simulink library "pmm"  (R2021b)
settings: Solver=VariableStepAuto  StartTime=0.0  StopTime=10.0  RelTol=1e-3
undefined symbols (not defined in the file or in its folder): ENUM_ACMAINRLYSTS_OPEN, ENUM_ACPRECHRGRLYSTS_OPEN, ENUM_B2VRLYSTA_OPEN, ENUM_BMSHVSTS_HVOPEN, ENUM_BRAKEPEDAL_RELEASED, ENUM_CACRLYDEM_CLOSE, ENUM_CACRLYSTS_OPEN, ENUM_CHRGFAULT_ACRLYFAIL, ENUM_CHRGFAULT_BCUHVFAIL, ENUM_CHRGFAULT_BCUNEGFAIL, ENUM_CHRGFAULT_BCUTIMEOUT, ENUM_CHRGFAULT_DCDCENABLE, ENUM_CHRGFAULT_DCDCRLYFAIL, ENUM_CHRGFAULT_HVILFAIL, ENUM_CHRGFAULT_PDUHVFAIL, ENUM_CHRGFAULT_RLYCHKFAIL, ENUM_DCDCEACPCURLYSTA_CLOSED, ENUM_DCDCEACPCURLYSTA_FAILTOCLOSE, ENUM_DCDCEACPCURLYSTA_OPEN, ENUM_DCDCEACPCURLYSTA_WELDED, ENUM_DCDCENABLESTS_READY, ENUM_DCDCRLYSTS_OPEN, ENUM_EHPSRLYDEM_CLOSE, ENUM_EHPSRLYSTS_OPEN, ENUM_FOGRLYENCMD_DISABLE, ENUM_GEARACTUALPOSN_D, ENUM_HVPWROFFREQ_POWEROFF, ENUM_KEYSTATUS_OFF, ENUM_KEYSTATUS_ON, ENUM_KEYSTATUS_START, ENUM_LOWBATTVOLTAGE_NORMAL, ENUM_LOWBATTVOLTAGE_POWERDOWN, ENUM_LOWBATTVOLTAGE_POWERUP, ENUM_MCUHVLOOP_POWEROFF, ENUM_MCUHVLOOPSTS_OPEN, ENUM_MCUMAINRLYSTS_OPEN, ENUM_MCUPRECHRGRLYSTS_OPEN, ENUM_PDFAULT_ACRLYOPEN, ENUM_PDFAULT_BCUDISABLE, ENUM_PDFAULT_DCDCDISABLE, ENUM_PDFAULT_DCDCRLYOPEN, ENUM_PDFAULT_EACDISABLE, ENUM_PDFAULT_EACRLYOPEN, ENUM_PDFAULT_EHPSDISABLE, ENUM_PDFAULT_EHPSRLYOPEN, ENUM_PDFAULT_MCUDISABLE, ENUM_PDFAULT_MCUDISCHRG, ENUM_PDFAULT_MCURLYOPEN, ENUM_PEUSELFCHKSTS_NOFAULT, ENUM_PLUGINSTS_NOPLUGIN, ENUM_PLUGINSTS_PLUGIN, ENUM_PMMMODE_DRIVE, ENUM_PMMMODE_LVBATCHRG, ENUM_PUSTATE_DCDCENABLE, ENUM_PUSTATE_EACPRESCHECK, ENUM_PUSTATE_EHPSENABLE, ENUM_PUSTATE_MCUENABLE, ENUM_PUSTATE_PDUMCURLYCLOSED, ENUM_PUSTATE_POWERUPFAIL, ENUM_TARGETGEAR_REVERSE ... (+126)
libraries: hcu_lib x45, simulink x5, ddm x1, dsc x1
(part 2 of 7)

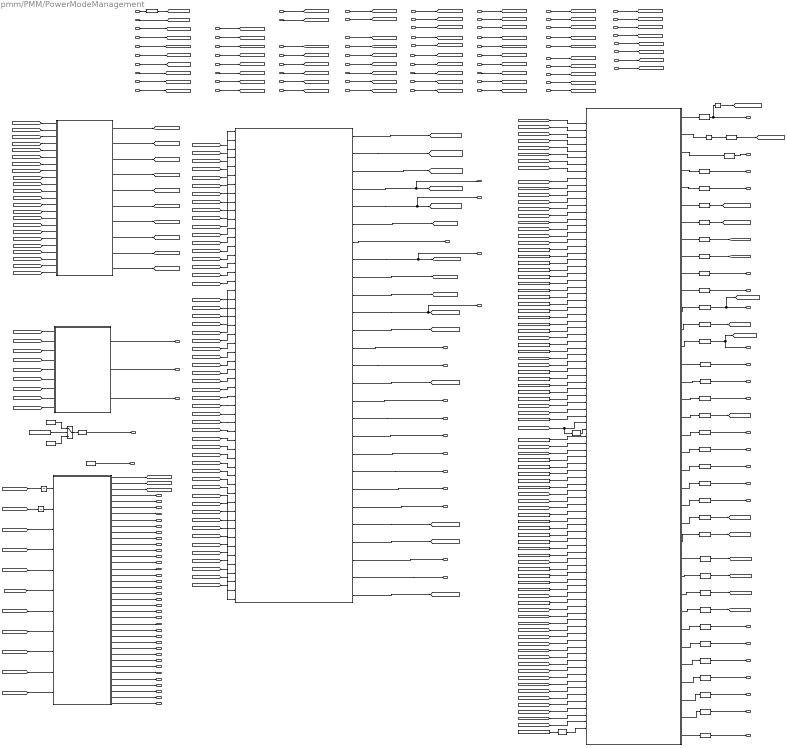
== system pmm/PMM/PowerModeManagement ==
  note: BDDM_outputs
  note: BDDM_outputs
  note: DDM_outpus
  note: BAPP_outputs
  note: BAPP_outputs
  note: BAPP_outputs
  note: BAPP_outputs
  note: BAPP_outputs
  note: BACC_outputs
  note: BVPSA_outputs
  task_time_s : Inport
  VPSA_Keystatus_enum : Inport  Port=2
  VPSA_EmergencyShutDown_flg : Inport  Port=3
  VPSA_AlcLockPass_flg : Inport  Port=4
  VACC_CACPresReady_flg : Inport  Port=5
  VTHC_AfterrunningMode_flg : Inport  Port=6
  VINP_DCChrgConnectSts_enum : Inport  Port=7
  VINP_BMSHVSts_enum : Inport  Port=8
  VINP_HVPwrOffReq_enum : Inport  Port=9
  VINP_MCUInVol_V : Inport  Port=10
  VINP_BMSChrgStatus_enum : Inport  Port=11
  VINP_B2VFaultCode_enum : Inport  Port=12
  VINP_AtvDisChgEnFbk_flg : Inport  Port=13
  VINP_MCUIGBTEnFbk_flg : Inport  Port=14
  VINP_MCUFailGrade_enum : Inport  Port=15
  VINP_MCUFailCode_enum : Inport  Port=16
  VINP_B2VHVILFault_flg : Inport  Port=17
  VINP_B2VMainNegRlySta_enum : Inport  Port=18
  VINP_B2VDCChgP1RlySta_enum : Inport  Port=19
  VINP_B2VDCChgN1RlySta_enum : Inport  Port=20
  VINP_B2VSOC_pct : Inport  Port=21
  VINP_MotorSpd_rpm : Inport  Port=22
  VINP_B2VPackCurr_A : Inport  Port=23
  VINP_B2VPackInsideVol_V : Inport  Port=24
  VINP_EACEnSta_enum : Inport  Port=25
  VINP_EHPSEnableStstus_enum : Inport  Port=26
  VINP_MCUHVLoopSts_enum : Inport  Port=27
  VINP_DCDCEnableStstus_enum : Inport  Port=28
  VINP_DCDCEnSta_enum : Inport  Port=29
  VINP_DCDCOutVol_V : Inport  Port=30
  VINP_PEUSelfChkSts_enum : Inport  Port=31
  VINP_MCUPrechrgRlySts_enum : Inport  Port=32
  VINP_HVILSta_enum : Inport  Port=33
  VINP_PDUMCUPosRlySta_enum : Inport  Port=34
  VINP_PDUACRlySta_enum : Inport  Port=35
  VINP_PDU3in1RlySta_enum : Inport  Port=36
  VINP_ParkBrakeSW_flg : Inport  Port=37
  VINP_EHPSMotorSpd_rpm : Inport  Port=38
  VINP_EBSBrakeSw_enum : Inport  Port=39
  VINP_TransReqGear_enum : Inport  Port=40
  VINP_ACPrechrgRlySts_enum : Inport  Port=41
  VINP_PushButton_flg : Inport  Port=42
  VINP_ChargeWakeup_flg : Inport  Port=43
  VINP_HVILPWMDuty_pct : Inport  Port=44
  VINP_VCUBattVol_v : Inport  Port=45
  VINP_MCUAfterRunReq_flg : Inport  Port=46
  VDSC_WineDetectorSwitch_flg : Inport  Port=47
  VDMM_LostComMCU_flg : Inport  Port=48
  VDMM_LostComPDU_flg : Inport  Port=49
  VDMM_LostComBCU : Inport  Port=50
  VDMM_LostComMCUSta2_flg : Inport  Port=51
  VDMM_RCIncorrect_flg : Inport  Port=52
  VDMM_DTCMCURCIncorrect_flg : Inport  Port=53
  VDMM_NoFeedBack_flg : Inport  Port=54
  VDMM_HVRlyNoFeedBack_flg : Inport  Port=55
  VDMM_DTCVCUPowerVolHigh_flg : Inport  Port=56
  VDMM_DTCVCUPowerVolLow_flg : Inport  Port=57
  VDMM_DTCHVILWireFailure_flg : Inport  Port=58
  VDMM_DTCAlcLockWireFailure_flg : Inport  Port=59
  VDMM_ProhibitCharge_flg : Inport  Port=60
  VDMM_ProhibitPowerUp_flg : Inport  Port=61
  VDMM_MCUForceDisable_flg : Inport  Port=62
  VDMM_DTCIRCS2GWireFailure_flg : Inport  Port=63
  VDMM_DTCIGNS2GWireFailure_flg : Inport  Port=64
  VDMM_DTCMCUCtrlMdNoFB_flg : Inport  Port=65
  VDMM_DTCBMSRlyNoFB_flg : Inport  Port=66
  VDMM_WireFailure_flg : Inport  Port=67
  VDIP_VCUVehSpd_kph : Inport  Port=68
  VTQD_GearActualPosn_enum : Inport  Port=69
  VTQD_LVchrgSvrMode_flg : Inport  Port=70
  VTQD_ActMDDoorOPSta_flg : Inport  Port=71
  VTQD_ActTDDoorOPSta_flg : Inport  Port=72
  VTQD_ActFRDoorOPSta_flg : Inport  Port=73
  Constant : Constant  Value=FALSE  OutDataTypeStr=boolean
  Constant1 : Constant  Value=KPMM_TimeHVSelfChk4Chrg_s
  Constant10 : Constant  Value=ZERO_INT
  Constant11 : Constant  Value=KPMM_Time4Sleep_s
  Constant12 : Constant  Value=KPMM_MCUPrechrgFailtime_s
  Constant13 : Constant  Value=KPMM_ForceEntrySleep_flg
  Constant14 : Constant  Value=KPMM_BCUGetChrgTO_s
  Constant15 : Constant  Value=KPMM_HVRlyOpenFailtime_s
  Constant16 : Constant  Value=KPMM_BattDownFailtime_s
  Constant17 : Constant  Value=KPMM_MCUDisChrgFailtime_s
  Constant18 : Constant  Value=KPMM_DCDCRlyDemDelayTime_s
  Constant19 : Constant  Value=KPMM_DCDCChrgFailtime_s
  Constant2 : Constant  Value=KPMM_SysInitialTO_s
  Constant20 : Constant  Value=KPMM_ChrgIntoPwrdownWait_s
  Constant21 : Constant  Value=KPMM_MCUEnDischrgFailtime_s
  Constant22 : Constant  Value=KPMM_TargetDchrgVolt_V
  Constant23 : Constant  Value=KPMM_TargetEnDischrgVolt_V
  Constant24 : Constant  Value=KPMM_HVRlyOpenFailWT_s
  Constant25 : Constant  Value=KPMM_WaitForAfterrunFail_s
  Constant26 : Constant  Value=KPMM_MCUPassDisChrg_s
  Constant27 : Constant  Value=KPMM_TargetPassDischrgVolt_V
  Constant28 : Constant  Value=KPMM_PDULoadRlyPUFailtime_s
  Constant29 : Constant  Value=KPMM_MCUEnableFailtime_s
  Constant3 : Constant  Value=KPMM_HVRlyCheckFailtime_s
  Constant30 : Constant  Value=KPMM_ForceMCUFailRst_flg
  Constant31 : Constant  Value=TRUE  OutDataTypeStr=boolean
  Constant32 : Constant  Value=KPMM_WaitAirPressTimeout_s
  Constant33 : Constant  Value=KPMM_AfterrunTimeout_s
  Constant34 : Constant  Value=KPSA_FakeWakeRESET_flg
  Constant4 : Constant  Value=KPMM_BattUpFailtime_s
  Constant45 : Constant  Value=KPMM_MCUDisChrgFSFailtime_s
  Constant46 : Constant  Value=KPMM_MCUDisableFailtime_s
  Constant47 : Constant  Value=KPMM_PDUDisableFailtime_s
  Constant48 : Constant  Value=KPMM_PDUDisableWaitime_s
  Constant5 : Constant  Value=KPMM_ButtonHoldlimit_cnt
  Constant59 : Constant  Value=KPMM_AlcLockCheckFailtime_s
  Constant6 : Constant  Value=KPMM_DCDCRlyUpFailtime_s
  Constant69 : Constant  Value=KPMM_EHPSEnTimout_s
  Constant7 : Constant  Value=KPMM_DCDCEnableFailtime_s
  Constant70 : Constant  Value=KPMM_EHPSIniTimout_s
  Constant71 : Constant  Value=KPMM_EHPSSpdDem_rpm
  Constant72 : Constant  Value=KPMM_EACEnTimout_s
  Constant8 : Constant  Value=KPMM_ChrgwakeDebon_cnt
  Constant9 : Constant  Value=KPMM_ACMainRlyUpFailtime_s
  Data Type Conversion : DataTypeConversion  OutDataTypeStr=single
  Data Type Conversion{1,3..5,10..12,25..26} (9 alike) : DataTypeConversion  OutDataTypeStr=uint8
  Data Type Conversion{2,6..7,13..17,22} (9 alike) : DataTypeConversion
  Data Type Conversion{8..9,18,20..21,23..24,27,31..37,39..40} (17 alike) : DataTypeConversion  OutDataTypeStr=boolean
  Data Type Conversion38 : DataTypeConversion  OutDataTypeStr=single
  Delay : Delay  DelayLength=1
  Delay1 : Delay  DelayLength=1
  Detect Increase : simulink/Logic and Bit Operations/Detect Increase  vinit=0.0  OutDataTypeStr=boolean
  Detect Increase1 : simulink/Logic and Bit Operations/Detect Increase  vinit=0.0  OutDataTypeStr=boolean
  Detect Increase2 : simulink/Logic and Bit Operations/Detect Increase  vinit=0.0  OutDataTypeStr=boolean
  "PMM " : Stateflow chart  Priority=2  TreatAsAtomicUnit=on
      settings: AttributesFormatString=< Priority = %<Priority>>  PortSchema="{\"entries\":[{\"content\":{\"sides\":[{\"content\":{\"connectorIds\":[\"In1\",\"In2\",\"In3\",\"In4\",\"In5\",\"In6\",\"In7\",\"In8\",\"In9\",\"In10\",\"In11\",\"In12\",\"In13\",\"In14\",\"In15\",\"In16\",\"In17\",\"In18\",\"In19\",\"In20\",\"In21\",\"In22\",\"In23\",\"In24\",\"In25\",\"In26\",\"In27\",\"In28\",\"In29\",\"In30\",\"In31\",\"In32\",\"In33\",\"In34\",\"In35\",\"In36\",\"In37\",\"In38\",\"In39\",\"In40\",\"In41\",\"In42\",\"In43\",\"In44\",\"In45\",\"In47\",\"In46\",\"In48\",\"In49\",\"In50\",\"In51\",\"In52\",\"In53\",\"In54\",\"In55\",\"In56\",\"In57\",\"In58\",\"In59\",\"In60\",\"In61\",\"In62\",\"In63\",\"In64\",\"In65\",\"In66\",\"In67\",\"In68\",\"In69\",\"In70\",\"In71\",\"In72\",\"In73\",\"In74\",\"In75\",\"In76\",\"In77\",\"In78\",\"In79\",\"In80\",\"In81\",\"In82\",\"In83\",\"In84\",\"In85\",\"In86\",\"In87\",\"In88\",\"In89\",\"In90\"]},\"type\":\"ConnectorPlacement.EquallySpacedRectSide\",\"uuid\":\"3283b3a6-ee09-4b30-80f8-87d8012d4677\"},{\"content\":{\"connectorIds\":[\"Out1\",\"Out2\",\"Out3\",\"Out4\",\"Out5\",\"Out6\",\"Out7\",\"Out8\",\"Out9\",\"Out10\",\"Out11\",\"Out12\",\"Out13\",\"Out14\",\"Out15\",\"Out16\",\"Out17\",\"Out18\",\"Out19\",\"Out20\",\"Out21\",\"Out22\",\"Out23\",\"Out24\",\"Out25\",\"Out26\",\"Out27\",\"Out28\",\"Out29\",\"Out30\",\"Out31\",\"Out32\",\"Out33\",\"Out34\",\"Out35\",\"Out36\"],\"side\":\"RIGHT\"},\"type\":\"ConnectorPlacement.EquallySpacedRectSide\",\"uuid\":\"c1188f1a-1dd1-4b88-b818-d9f7ca918d77\"},{\"content\":{\"connectorIds\":[],\"side\":\"TOP\"},\"type\":\"ConnectorPlacement.EquallySpacedRectSide\",\"uuid\":\"5e968c55-6da2-4142-9dc8-82ede108025c\"},{\"content\":{\"connectorIds\":[],\"side\":\"HIDDEN\"},\"type\":\"ConnectorPlacement.EquallySpacedRectSide\",\"uuid\":\"849a9414-5dfb-49c9-9dd5-bd25908a36e0\"}]},\"type\":\"ConnectorPlacement.EquallySpacedConnector\",\"uuid\":\"326bbf94-b030-4298-91d3-64ac1e293607\"}],\"packageUris\":[\"http://schema.mathworks.com/mf0/Connector/R2020b\"],\"version\":\"1.0\"}"
  "PMM Flag Creator " : Subsystem
  PMM State Change Configuration : Subsystem
  PMM Switch Enum Creator : Subsystem
  PMM_SCP : Subsystem  TreatAsAtomicUnit=on
      settings: RTWSystemCode=Nonreusable function  RTWFcnNameOpts=Use subsystem name  RTWFileNameOpts=Use subsystem name
  Switch : Switch  Criteria=u2 > Threshold
  Unit Delay : UnitDelay  SampleTime=-1  HasFrameUpgradeWarning=on
  Unit Delay1 : UnitDelay  SampleTime=-1  HasFrameUpgradeWarning=on
  VPMM_SysPowerMode_enum : Outport  VectorParamsAs1DForOutWhenUnconnected=off
  VPMM_PowerUpState_enum : Outport  Port=2  VectorParamsAs1DForOutWhenUnconnected=off
  VPMM_PowerDownState_enum : Outport  Port=3  VectorParamsAs1DForOutWhenUnconnected=off
  VPMM_ChrgState_enum : Outport  Port=4  VectorParamsAs1DForOutWhenUnconnected=off
  VPMM_PowerUpFault_enum : Outport  Port=5  VectorParamsAs1DForOutWhenUnconnected=off
  VPMM_PowerDownFault_enum : Outport  Port=6  VectorParamsAs1DForOutWhenUnconnected=off
  VPMM_ChrgFault_enum : Outport  Port=7  VectorParamsAs1DForOutWhenUnconnected=off
  VPMM_IRCRlyClose_flg : Outport  Port=8  VectorParamsAs1DForOutWhenUnconnected=off
  VPMM_IGNRlyClose_flg : Outport  Port=9  VectorParamsAs1DForOutWhenUnconnected=off
  VPMM_BattHVDem_enum : Outport  Port=10  VectorParamsAs1DForOutWhenUnconnected=off
  VPMM_DCDCRlyDem_enum : Outport  Port=11  VectorParamsAs1DForOutWhenUnconnected=off
  VPMM_CACRlyDem_enum : Outport  Port=12  VectorParamsAs1DForOutWhenUnconnected=off
  VPMM_MCUHVLoopDem_enum : Outport  Port=13  VectorParamsAs1DForOutWhenUnconnected=off
  VPMM_EHPSR lyDem_enum : Outport  Port=14  VectorParamsAs1DForOutWhenUnconnected=off
  VPMM_ACHVLoopDem_enum : Outport  Port=15  VectorParamsAs1DForOutWhenUnconnected=off
  VPMM_HVSysReady_enum : Outport  Port=16  VectorParamsAs1DForOutWhenUnconnected=off
  VPMM_DrivelineRelease_enum : Outport  Port=17  VectorParamsAs1DForOutWhenUnconnected=off
  VPMM_PMMDCDCEnableDem_flg : Outport  Port=18  VectorParamsAs1DForOutWhenUnconnected=off
  VPMM_ActiveDischargeReq_enum : Outport  Port=19  VectorParamsAs1DForOutWhenUnconnected=off
  VPMM_PowerDownCompleted_flg : Outport  Port=20  VectorParamsAs1DForOutWhenUnconnected=off
  VPMM_PowerUpComplete_flg : Outport  Port=21  VectorParamsAs1DForOutWhenUnconnected=off
  VPMM_ExtTorquePrevent_enum : Outport  Port=22  VectorParamsAs1DForOutWhenUnconnected=off
  VPMM_PowerUpInhibit_flg : Outport  Port=23  VectorParamsAs1DForOutWhenUnconnected=off
  VPMM_VCUMCUEn_flg : Outport  Port=24  VectorParamsAs1DForOutWhenUnconnected=off
  VPMM_VCUMCUCtrlMd_enum : Outport  Port=25  VectorParamsAs1DForOutWhenUnconnected=off
  VPMM_VCUMCUFailRst_flg : Outport  Port=26  VectorParamsAs1DForOutWhenUnconnected=off
  VPMM_HVILFail_flg : Outport  Port=27  VectorParamsAs1DForOutWhenUnconnected=off
  VPMM_PMMEACEnableDem_flg : Outport  Port=28
  VPMM_PMMEHPSDemSpd_rpm : Outport  Port=29
  VPMM_PMMEHPSEnableDem_flg : Outport  Port=30
  VPMM_EHPSIniFinish_flg : Outport  Port=31
  VPMM_EACEnableCompleted_flg : Outport  Port=32
  VPMM_AlcLockSta_flg : Outport  Port=33  VectorParamsAs1DForOutWhenUnconnected=off
  VPMM_LostHVComActivePwrDown_flg : Outport  Port=34  VectorParamsAs1DForOutWhenUnconnected=off
  VPMM_LVBattLowInd_flg : Outport  Port=35  VectorParamsAs1DForOutWhenUnconnected=off
  VPMM_ChrgPowerUpFail_flg : Outport  Port=36
  VPMM_ChrgBCUHVFail_flg : Outport  Port=37
  VPMM_HVFailureChkPass_flg : Outport  Port=38  VectorParamsAs1DForOutWhenUnconnected=off
  VPMM_HVILDetectFail_flg : Outport  Port=39  VectorParamsAs1DForOutWhenUnconnected=off
  VPMM_LVChrgPreActFinished_flg : Outport  Port=40  VectorParamsAs1DForOutWhenUnconnected=off
  VPMM_TrigRBuzeer_flg : Outport  Port=41  VectorParamsAs1DForOutWhenUnconnected=off
  VPMM_TrigRLamp_flg : Outport  Port=42  VectorParamsAs1DForOutWhenUnconnected=off
  VPMM_TrigBrkLamp_flg : Outport  Port=43  VectorParamsAs1DForOutWhenUnconnected=off
  VPMM_DCDCVolLowTO_flg : Outport  Port=44  VectorParamsAs1DForOutWhenUnconnected=off
  VPMM_LongIdleDetFinsh_flg : Outport  Port=45  VectorParamsAs1DForOutWhenUnconnected=off
  VPMM_V2BLifeSig_cnt : Outport  Port=46
  VPMM_V2BAux1OnOff_enum : Outport  Port=47
  VPMM_V2BAux2OnOff_enum : Outport  Port=48
  VPMM_V2BAux3OnOff_enum : Outport  Port=49
  VPMM_V2BMainPosRlySta_enum : Outport  Port=50
  VPMM_V2BMainPosRlyFit_enum : Outport  Port=51
  VPMM_V2BACPosRlySta_enum : Outport  Port=52
  VPMM_V2BACPosRlyFit_enum : Outport  Port=53
  VPMM_V2BAirPosRlySta_enum : Outport  Port=54
  VPMM_V2BAirPosRlyFit_enum : Outport  Port=55
  VPMM_V2BOilrPosRlySta_enum : Outport  Port=56
  VPMM_V2BOilPosRlyFit_enum : Outport  Port=57
  VPMM_V2BDCDCPosRlySta_enum : Outport  Port=58
  VPMM_V2BDCDCPosRlyFit_enum : Outport  Port=59
  VPMM_V2BAux1RlySta_enum : Outport  Port=60
  VPMM_V2BAux1RlyFit_enum : Outport  Port=61
  VPMM_V2BAux2RlySta_enum : Outport  Port=62
  VPMM_V2BAux2RlyFit_enum : Outport  Port=63
  VPMM_V2BAux3RlySta_enum : Outport  Port=64
  VPMM_V2BAux3RlyFit_enum : Outport  Port=65
  VPMM_V2BAux4RlySta_enum : Outport  Port=66
  VPMM_V2BAux4RlyFit_enum : Outport  Port=67
  VPMM_V2BRsv1_cnt : Outport  Port=68
  VPMM_V2BRsv2_cnt : Outport  Port=69
  VPMM_VCULife1_cnt : Outport  Port=70
  VPMM_VCULife2_cnt : Outport  Port=71
  VPMM_VSPFunc_enum : Outport  Port=72
  VPMM_VSPIGNKeySta_enum : Outport  Port=73
  VPMM_VSPReversed_flg : Outport  Port=74
  VPMM_VSPTurnRight_enum : Outport  Port=75
  VPMM_VSPTurnLeft_enum : Outport  Port=76
  VPMM_FogTMSRlyCMD_enum : Outport  Port=77  VectorParamsAs1DForOutWhenUnconnected=off
  VPMM_DCCurr_A : Outport  Port=78  VectorParamsAs1DForOutWhenUnconnected=off
  VPMM_DCVol_V : Outport  Port=79  VectorParamsAs1DForOutWhenUnconnected=off
  wires:
  VTQD_LVchrgSvrMode_flg/1 -> [VSCP_LVchrgSvrMode_flg]
  "PMM Flag Creator "/18(VPMM_HVILDetectFail_flg) -> VPMM_HVILDetectFail_flg/1
  [VINP_MCUFailCode_enum] -> "PMM Flag Creator "/12(VINP_MCUFailCode_enum)
  [VINP_HVPwrOffReq_enum] -> "PMM Flag Creator "/19(VINP_HVPwrOffReq_enum)
  [VINP_B2VFaultCode_enum] -> "PMM Flag Creator "/14(VINP_B2VFaultCode_enum)
  [VDIP_VCUVehSpd_kph] -> "PMM Flag Creator "/31(VDIP_VCUVehSpd_kph)
  [VPMM_PDUEHPSRlySta_enum] -> "PMM Flag Creator "/6(VSCP_PDUEHPSRlySta_enum)
  [VINP_B2VDCChgN1RlySta_enum] -> "PMM Flag Creator "/17(VINP_B2VDCChgN1RlySta_enum)
  [VINP_B2VDCChgP1RlySta_enum] -> "PMM Flag Creator "/16(VINP_B2VDCChgP1RlySta_enum)
  [VPMM_MCUEnableProc_flg] -> PMM Switch Enum Creator/4(VPMM_MCUEnableProc_flg)
  [VPMM_MCUPrechrgProc_flg] -> PMM Switch Enum Creator/3(VPMM_MCUPrechrgProc_flg)
  [VDMM_RCIncorrect_flg] -> "PMM Flag Creator "/34(VDMM_RCIncorrect_flg)
  "PMM Flag Creator "/12(VPMM_RCIncorrect_flg) -> [VPMM_RCIncorrect_flg]
  [task_time_s] -> "PMM Flag Creator "/1(task_time_s)
  [VINP_B2VMainNegRlySta_enum] -> "PMM Flag Creator "/15(VINP_B2VMainNegRlySta_enum)
  [VDMM_LostComMCU_flg] -> "PMM Flag Creator "/32(VDMM_LostComMCU_flg)
  [VPMM_IRCRlyClose_flg] -> "PMM Flag Creator "/20(VPMM_IRCRlyClose_flg)
  [VPMM_PDUDCDCRlySta_enum] -> "PMM Flag Creator "/5(VSCP_PDUDCDCRlySta_enum)
  [VINP_EHPSMotorSpd_rpm] -> "PMM Flag Creator "/25(VINP_EHPSMotorSpd_rpm)
  [VINP_PDUACRlySta_enum] -> "PMM Flag Creator "/9(VINP_PDUACRlySta_enum)
  "PMM Flag Creator "/2(VPMM_HVUnitSelfChkCompleted4PU_flg) -> [VPMM_HVUnitSelfChkCompleted4PU_flg]
  [VPMM_LVChrgPreActFinished_flg] -> PMM State Change Configuration/3(VPMM_DCDCVolLowTO_flg)
  PMM State Change Configuration/8(VPMM_Charge2PowerDown_flg) -> [VPMM_Charge2PowerDown_flg]
  [VPMM_HVILFail_flg] -> PMM State Change Configuration/5(VPMM_HVILEmergencyStop_flg)
  [VINP_B2VHVILFault_flg] -> "PMM Flag Creator "/13(VINP_B2VHVILFault_flg)
  [VINP_DCChrgConnectSts_enum] -> PMM State Change Configuration/4(VINP_DCChrgConnectSts_enum)
  PMM State Change Configuration/5(VPMM_Initialize2PowerUp_flg) -> [VPMM_Initialize2PowerUp_flg]
  PMM State Change Configuration/2(VPMM_AfterRun2Initialize_flg) -> [VPMM_AfterRun2Initialize_flg]
  PMM State Change Configuration/1(VPMM_Boot2Initialize_flg) -> [VPMM_Boot2Initialize_flg]
  "PMM Flag Creator "/7(VPMM_LVBattLowInd_flg) -> VPMM_LVBattLowInd_flg/1
  [VPSA_EmergencyShutDown_flg] -> PMM State Change Configuration/6(VPSA_EmergencyShutDown_flg)
  "PMM Flag Creator "/9(VPMM_MCUSta2Lost_flg) -> [VPMM_MCUSta2Lost_flg]
  "PMM Flag Creator "/8(VPMM_LVChrgPreActFinished_flg) -> VPMM_LVChrgPreActFinished_flg/1, [VPMM_LVChrgPreActFinished_flg]
  "PMM Flag Creator "/4(VPMM_HVFailureChkPass_flg) -> VPMM_HVFailureChkPass_flg/1, [VPMM_HVFailureChkPass_flg]
  "PMM Flag Creator "/3(VPMM_HVUnitSelfChkCompleted4Chrg_flg) -> [VPMM_HVUnitSelfChkCompleted4Chrg_flg]
  [VPMM_LostHVComActivePwrDown_flg] -> PMM State Change Configuration/7(VPMM_LostCom_flg)
  PMM State Change Configuration/7(VPMM_Drive2PowerDown_flg) -> [VPMM_Drive2PowerDown_flg]
  [VDMM_LostComMCUSta2_flg] -> "PMM Flag Creator "/28(VDMM_LostComMCUSta2_flg)
  [VDMM_LostComPDU_flg] -> "PMM Flag Creator "/33(VDMM_LostComPDU_flg)
  PMM Switch Enum Creator/2(VPMM_PowerDownFault_enum) -> VPMM_PowerDownFault_enum/1
  [VPMM_PowerUpState_enum] -> PMM Switch Enum Creator/1(VPMM_InitPowerUpState_enum)
  VINP_B2VMainNegRlySta_enum/1 -> [VINP_B2VMainNegRlySta_enum]
  VTHC_AfterrunningMode_flg/1 -> [VTHC_AfterrunningMode_flg]
  VINP_MCUIGBTEnFbk_flg/1 -> [VINP_MCUIGBTEnFbk_flg]
  VINP_MCUInVol_V/1 -> [VINP_MCUInVol_V]
  VINP_MCUAfterRunReq_flg/1 -> [VINP_MCUAfterRunReq_flg]
  VINP_EACEnSta_enum/1 -> [VINP_EACEnSta_enum]
  [VPMM_IGNRlyClose_flg] -> "PMM Flag Creator "/21(VPMM_IGNRlyClose_flg)
  VINP_DCChrgConnectSts_enum/1 -> [VINP_DCChrgConnectSts_enum]
  PMM Switch Enum Creator/3(VPMM_ChrgFault_enum) -> VPMM_ChrgFault_enum/1
  [VINP_HVILPWMDuty_pct] -> "PMM Flag Creator "/22(VINP_HVILPWMDuty_pct)
  VINP_MCUPrechrgRlySts_enum/1 -> [VINP_MCUPrechrgRlySts_enum]
  VINP_AtvDisChgEnFbk_flg/1 -> [VINP_AtvDisChgEnFbk_flg]
  VINP_MCUFailCode_enum/1 -> [VINP_MCUFailCode_enum]
  VINP_DCDCOutVol_V/1 -> [VINP_DCDCOutVol_V]
  VPSA_Keystatus_enum/1 -> [VPSA_Keystatus_enum]
  VINP_B2VDCChgP1RlySta_enum/1 -> [VINP_B2VDCChgP1RlySta_enum]
  task_time_s/1 -> Data Type Conversion/1
  VINP_HVPwrOffReq_enum/1 -> [VINP_HVPwrOffReq_enum]
  VDMM_DTCMCURCIncorrect_flg/1 -> [VDMM_DTCMCURCIncorrect_flg]
  VINP_BMSChrgStatus_enum/1 -> [VINP_BMSChrgStatus_enum]
  VINP_ChargeWakeup_flg/1 -> [VINP_ChargeWakeup_flg]
  VINP_BMSHVSts_enum/1 -> [VINP_BMSHVSts_enum]
  VINP_HVILPWMDuty_pct/1 -> [VINP_HVILPWMDuty_pct]
  VPSA_EmergencyShutDown_flg/1 -> [VPSA_EmergencyShutDown_flg]
  VINP_EHPSEnableStstus_enum/1 -> [VINP_EHPSEnableStstus_enum]
  VDIP_VCUVehSpd_kph/1 -> [VDIP_VCUVehSpd_kph]
  Data Type Conversion/1 -> [task_time_s]  "task_time_s"
  VDSC_WineDetectorSwitch_flg/1 -> [VDSC_WineDetectorSwitch_flg]
  VINP_PushButton_flg/1 -> [VINP_PushButton_flg]
  VDMM_LostComMCU_flg/1 -> [VDMM_LostComMCU_flg]
  "PMM Flag Creator "/6(VPMM_EHPSIniReady_flg) -> [VPMM_EHPSIniReady_flg]
  VDMM_LostComBCU/1 -> [VDMM_LostComBCU]
  VACC_CACPresReady_flg/1 -> [VACC_CACPresReady_flg]
  VINP_B2VFaultCode_enum/1 -> [VINP_B2VFaultCode_enum]
  VINP_B2VHVILFault_flg/1 -> [VINP_B2VHVILFault_flg]
  [VINP_ACPrechrgRlySts_enum] -> "PMM Flag Creator "/8(VINP_ACPrechrgRlySts_enum)
  VINP_PDUACRlySta_enum/1 -> [VINP_PDUACRlySta_enum]
  [VDSC_WineDetectorSwitch_flg] -> "PMM Flag Creator "/24(VDSC_WineDetectorSwitch_flg)
  [VINP_DCDCOutVol_V] -> "PMM Flag Creator "/26(VINP_DCDCOutVol_V)
  VINP_EHPSMotorSpd_rpm/1 -> [VINP_EHPSMotorSpd_rpm]
  [VPMM_ChrgFault_enum] -> PMM Switch Enum Creator/9(VPMM_InitChrgFault_enum)
  [VINP_PEUSelfChkSts_enum] -> "PMM Flag Creator "/10(VINP_PEUSelfChkSts_enum)
  [VPMM_MCUHVLoopDem_enum] -> "PMM Flag Creator "/37(VPMM_InitMCUHVLoopDem_enum)
  [VDMM_LostComBCU] -> "PMM Flag Creator "/30(VDMM_LostComBCU)
  [VINP_MCUPrechrgRlySts_enum] -> "PMM Flag Creator "/3(VINP_MCUPrechrgRlySts_enum)
  [VINP_MCUFailGrade_enum] -> "PMM Flag Creator "/11(VINP_MCUFailGrade_enum)
  "PMM Flag Creator "/13(VPMM_VCUMCUEn_flg) -> VPMM_VCUMCUEn_flg/1
  [VPMM_DCDCEnableProc_flg] -> PMM Switch Enum Creator/5(VPMM_DCDCEnableProc_flg)
  Constant19/1 -> "PMM "/27(KPMM_DCDCChrgFailtime_s)
  Data Type Conversion14/1 -> [VPMM_EHPSRlyDem_enum], VPMM_EHPSR lyDem_enum/1  "VPMM_EHPSRlyDem_enum"
  [VPMM_CACPresReadyProc_flg] -> PMM Switch Enum Creator/7(VPMM_CACPresReadyProc_flg)
  Detect Increase/1 -> VPMM_VCUMCUFailRst_flg/1  "VPMM_VCUMCUFailRst_flg"
  VINP_B2VDCChgN1RlySta_enum/1 -> [VINP_B2VDCChgN1RlySta_enum]
  "PMM "/4(VPMM_ChrgState_enum) -> Data Type Conversion4/1
  [VINP_BMSHVSts_enum] -> "PMM "/4(VINP_BMSHVSts_enum)
  PMM State Change Configuration/4(VPMM_Initialize2Charge_flg) -> [VPMM_Initialize2Charge_flg]
  "PMM "/6(VPMM_PowerDownFault_enum) -> Data Type Conversion6/1
  "PMM "/13(VPMM_MCUHVLoopDem_enum) -> Data Type Conversion13/1
  Constant20/1 -> "PMM "/59(KPMM_ChrgIntoPwrdownWait_s)
  "PMM "/12(VPMM_CACRlyDem_enum) -> Data Type Conversion12/1
  [VDMM_DTCMCURCIncorrect_flg] -> "PMM Flag Creator "/35(VDMM_DTCMCURCIncorrect_flg)
  [VINP_MCUFailGrade_enum] -> "PMM "/36(VINP_MCUFailGrade_enum)
  VINP_DCDCEnSta_enum/1 -> [VINP_DCDCEnSta_enum]
  "PMM "/21(VPMM_PowerUpComplete_flg) -> Data Type Conversion24/1
  "PMM "/15(VPMM_ACHVLoopDem_enum) -> Data Type Conversion15/1
  Constant27/1 -> "PMM "/54(KPMM_TargetPassDischrgVolt_V)
  Data Type Conversion27/1 -> [VPMM_VCUMCUEn_flg]  "VPMM_VCUMCUEn_flg"
  Constant45/1 -> "PMM "/61(KPMM_MCUDisChrgFSFailtime_s)
  "PMM "/19(VPMM_PowerUpInhibit_flg) -> Data Type Conversion22/1
  Constant6/1 -> "PMM "/21(KPMM_DCDCRlyUpFailtime_s)
  [VINP_MCUHVLoopSts_enum] -> "PMM Flag Creator "/18(VINP_MCUHVLoopSts_enum)
  "PMM "/30(VPMM_PMMEACEnableDem_flg) -> Data Type Conversion37/1
  Constant/1 -> Switch/3
  [VINP_MCUAfterRunReq_flg] -> "PMM "/17(VINP_MCUAfterRunReq_flg)
  Data Type Conversion9/1 -> [VPMM_IGNRlyClose_flg]  "VPMM_IGNRlyClose_flg"
  PMM State Change Configuration/6(VPMM_PowerUp2PowerDown_flg) -> [VPMM_PowerUp2PowerDown_flg]
  Data Type Conversion3/1 -> VPMM_PowerDownState_enum/1  "VPMM_PowerDownState_enum"
  [VINP_MCUIGBTEnFbk_flg] -> "PMM "/18(VINP_MCUIGBTEnFbk_flg)
  [VINP_PEUSelfChkSts_enum] -> "PMM "/56(VINP_PEUSelfChkSts_enum)
  PMM State Change Configuration/3(VPMM_Initialize2Idle_flg) -> [VPMM_Initialize2Idle_flg]
  [VPMM_AtvDisChgEnFbk_flg] -> "PMM "/73(VPMM_AtvDisChgEnFbk_flg)
  Data Type Conversion8/1 -> [VPMM_IRCRlyClose_flg]  "VPMM_IRCRlyClose_flg"
  Data Type Conversion15/1 -> VPMM_ACHVLoopDem_enum/1  "VPMM_ACHVLoopDem_enum"
  "PMM "/17(VPMM_DrivelineRelease_enum) -> Data Type Conversion17/1
  "PMM "/9(VPMM_IGNRlyClose_flg) -> Data Type Conversion9/1
  Data Type Conversion31/1 -> [VPMM_MCUPrechrgProc_flg]  "VPMM_MCUPrechrgProc_flg"
  Data Type Conversion12/1 -> [VPMM_CACRlyDem_enum], VPMM_CACRlyDem_enum/1  "VPMM_CACRlyDem_enum"
  [VPMM_PDUEACRlySta_enum] -> "PMM "/8(VPMM_PDUEACRlySta_enum)
  [VINP_MCUHVLoopSts_enum] -> "PMM "/9(VINP_MCUHVLoopSts_enum)
  PMM Switch Enum Creator/1(VPMM_PowerUpState_enum) -> VPMM_PowerUpState_enum/1
  Constant48/1 -> "PMM "/64(KPMM_PDUDisableWaitime_s)
  Data Type Conversion13/1 -> [VPMM_MCUHVLoopDem_enum]  "VPMM_MCUHVLoopDem_enum"
  "PMM Flag Creator "/1(VPMM_RlyOpenCheck_flg) -> [VPMM_RlyOpenCheck_flg]
  "PMM "/14(VPMM_EHPSRlyDem_enum) -> Data Type Conversion14/1
  Constant33/1 -> "PMM "/41(KPMM_AfterrunTimeout_s)
  "PMM "/34(VPMM_EACEnableCompleted_flg) -> Data Type Conversion36/1
  Constant32/1 -> "PMM "/40(KPMM_WaitAirPressTimeout_s)
  [VPMM_HVILFail_flg] -> "PMM "/42(VPMM_HVILEmergencyStop_flg)
  [VPSA_Keystatus_enum] -> "PMM "/2(VPSA_Keystatus_enum)
  "PMM "/27(VPMM_DCDCEnableProc_flg) -> Data Type Conversion33/1
  Constant8/1 -> "PMM "/46(KPMM_ChrgwakeDebon_cnt)
  Constant10/1 -> VPMM_ActiveDischargeReq_enum/1  "VPMM_ActiveDischargeReq_enum"
  [task_time_s] -> PMM Switch Enum Creator/2(task_time_s)
  "PMM "/32(VPMM_PMMEHPSEnableDem_flg) -> Data Type Conversion39/1
  VINP_DCDCEnableStstus_enum/1 -> [VINP_DCDCEnableStstus_enum]
  Data Type Conversion16/1 -> VPMM_HVSysReady_enum/1  "VPMM_HVSysReady_enum"
  Data Type Conversion1/1 -> Delay/1, VPMM_SysPowerMode_enum/1  "VPMM_SysPowerMode_enum"
  Data Type Conversion23/1 -> VPMM_PowerDownCompleted_flg/1  "VPMM_PowerDownCompleted_flg"
  Data Type Conversion26/1 -> VPMM_VCUMCUCtrlMd_enum/1  "VPMM_VCUMCUCtrlMd_enum"
  "PMM "/33(VPMM_EHPSIniFinish_flg) -> Data Type Conversion21/1
  VINP_HVILSta_enum/1 -> [VINP_HVILSta_enum]
  [VPSA_AlcLockPass_flg] -> "PMM "/65(VPSA_AlcLockPass_flg)
  "PMM "/25(VPMM_MCUPrechrgProc_flg) -> Data Type Conversion31/1
  VINP_ACPrechrgRlySts_enum/1 -> [VINP_ACPrechrgRlySts_enum]
  [VPMM_MCUSta2Lost_flg] -> "PMM "/72(VPMM_MCUSta2Lost_flg)
  Data Type Conversion10/1 -> VPMM_BattHVDem_enum/1  "VPMM_BattHVDem_enum"
  [VPSA_Keystatus_enum] -> PMM State Change Configuration/1(VPSA_Keystatus_enum)
  Data Type Conversion21/1 -> VPMM_EHPSIniFinish_flg/1  "VPMM_EHPSIniFinish_flg"
  "PMM "/36(VPMM_ChrgBCUHVFail_flg) -> Data Type Conversion40/1
  "PMM "/31(VPMM_PMMEHPSDemSpd_rpm) -> Data Type Conversion38/1
  Data Type Conversion38/1 -> VPMM_PMMEHPSDemSpd_rpm/1  "VPMM_PMMEHPSDemSpd_rpm"
  Data Type Conversion33/1 -> [VPMM_DCDCEnableProc_flg]  "VPMM_DCDCEnableProc_flg"
  Data Type Conversion2/1 -> [VPMM_PowerUpState_enum]  "VPMM_PowerUpState_enum"
  Data Type Conversion5/1 -> VPMM_PowerUpFault_enum/1  "VPMM_PowerUpFault_enum"
  [VPMM_HVFailureChkPass_flg] -> "PMM "/55(VPMM_HVFailureChkPass_flg)
  Data Type Conversion32/1 -> [VPMM_MCUEnableProc_flg]  "VPMM_MCUEnableProc_flg"
  Constant69/1 -> "PMM "/67(KPMM_EHPSENTimeout_s)
  [VPMM_VCUMCUEn_flg] -> "PMM Flag Creator "/36(VPMM_InitVCUMCUEn_flg)
  Data Type Conversion36/1 -> VPMM_EACEnableCompleted_flg/1  "VPMM_EACEnableCompleted_flg"
  "PMM "/3(VPMM_PowerDownState_enum) -> Data Type Conversion3/1
  Constant14/1 -> "PMM "/58(KPMM_BCUGetChrgTO_s)
  Constant47/1 -> "PMM "/63(KPMM_PDUDisableFailtime_s)
  Constant72/1 -> "PMM "/71(KPMM_EACENTimeout_s)
  "PMM "/20(VPMM_PowerDownCompleted_flg) -> Data Type Conversion23/1
  Data Type Conversion20/1 -> VPMM_ChrgPowerUpFail_flg/1  "VPMM_ChrgPowerUpFail_flg"
  Constant26/1 -> "PMM "/53(KPMM_MCUPassDisChrg_s)
  "PMM "/16(VPMM_HVSysReady_enum) -> Data Type Conversion16/1
  [VPMM_EHPSEnableProc_flg] -> PMM Switch Enum Creator/6(VPMM_EHPSEnableProc_flg)
  VINP_MCUHVLoopSts_enum/1 -> [VINP_MCUHVLoopSts_enum]
  [VPMM_RCIncorrect_flg] -> PMM State Change Configuration/8(VPMM_RCIncorrect_flg)
  Constant15/1 -> "PMM "/50(KPMM_HVRlyOpenFailtime_s)
  Data Type Conversion40/1 -> VPMM_ChrgBCUHVFail_flg/1  "VPMM_ChrgBCUHVFail_flg"
  [VPMM_PowerDownFault_enum] -> PMM Switch Enum Creator/8(VPMM_InitPowerDownFault_enum)
  Data Type Conversion17/1 -> VPMM_DrivelineRelease_enum/1  "VPMM_DrivelineRelease_enum"
  [VINP_PDUMCUPosRlySta_enum] -> "PMM "/48(VINP_PDUMCUPosRlySta_enum)
  [VINP_AtvDisChgEnFbk_flg] -> "PMM Flag Creator "/29(VINP_AtvDisChgEnFbk_flg)
  "PMM Flag Creator "/11(VPMM_LostHVComActivePwrDown_flg) -> [VPMM_LostHVComActivePwrDown_flg], VPMM_LostHVComActivePwrDown_flg/1
  Data Type Conversion37/1 -> VPMM_PMMEACEnableDem_flg/1  "VPMM_PMMEACEnableDem_flg"
  Constant1/1 -> "PMM "/29(KPMM_TimeHVSelfChk4Chrg_s)
  Data Type Conversion18/1 -> [VPMM_DCDCEnableDem_flg]  "VPMM_DCDCEnableDem_flg"
  Constant30/1 -> Switch/2
  Constant21/1 -> "PMM "/51(KPMM_MCUEnDischrgFailtime_s)
  "PMM "/29(VPMM_CACPresReadyProc_flg) -> Data Type Conversion35/1
  Constant5/1 -> "PMM "/44(KPMM_ButtonHoldlimit_cnt)
  [VINP_EACEnSta_enum] -> "PMM "/12(VINP_EACEnSta_enum)
  "PMM "/26(VPMM_MCUEnableProc_flg) -> Data Type Conversion32/1
  "PMM "/18(VPMM_PMMDCDCEnableDem_flg) -> Data Type Conversion18/1
  Constant11/1 -> "PMM "/33(KPMM_Time4Sleep_s)
  [VINP_PDUMCUPosRlySta_enum] -> "PMM Flag Creator "/2(VINP_PDUMCUPosRlySta_enum)
  [VINP_HVILSta_enum] -> "PMM Flag Creator "/23(VINP_HVILSta_enum)
  Constant28/1 -> "PMM "/39(KPMM_PDULoadRlyPUFailtime_s)
  [VTHC_AfterrunningMode_flg] -> "PMM "/43(VTHC_AfterrunningMode_flg)
  Constant3/1 -> "PMM "/19(KPMM_HVRlyCheckFailtime_s)
  Constant29/1 -> "PMM "/37(KPMM_MCUEnableFailtime_s)
  "PMM "/1(VPMM_SysPowerMode_enum) -> Data Type Conversion1/1
  VINP_PEUSelfChkSts_enum/1 -> [VINP_PEUSelfChkSts_enum]
  Constant13/1 -> "PMM "/34(KPMM_ForceEntrySleep_flg)
  "PMM Flag Creator "/5(VPMM_HVILFail_flg) -> VPMM_HVILFail_flg/1, [VPMM_HVILFail_flg]
  Constant24/1 -> "PMM "/60(KPMM_HVRlyOpenFailWT_s)
  "PMM "/24(VPMM_VCUMCUEn_flg) -> Data Type Conversion27/1
  VDMM_RCIncorrect_flg/1 -> [VDMM_RCIncorrect_flg]
  Data Type Conversion7/1 -> [VPMM_ChrgFault_enum]
  [VPMM_PDUEHPSRlySta_enum] -> "PMM "/7(VPMM_PDUEHPSRlySta_enum)
  VDMM_LostComPDU_flg/1 -> [VDMM_LostComPDU_flg]
  [VINP_MCUInVol_V] -> "PMM "/13(VINP_MCUInVol_V)
  "PMM Flag Creator "/10(VPMM_AtvDisChgEnFbk_flg) -> [VPMM_AtvDisChgEnFbk_flg]
  [VPMM_HVUnitSelfChkCompleted4PU_flg] -> "PMM "/32(VPMM_HVUnitSelfChkCompleted4PU_flg)
  [VPMM_EHPSIniReady_flg] -> "PMM "/70(VPMM_EHPSIniReady_flg)
  Constant70/1 -> "PMM "/68(KPMM_EHPSIniTimeout_s)
  Data Type Conversion6/1 -> [VPMM_PowerDownFault_enum]
  Constant12/1 -> "PMM "/24(KPMM_MCUPrechrgFailtime_s)
  [VINP_DCDCEnSta_enum] -> "PMM Flag Creator "/27(VINP_DCDCEnSta_enum)
  "PMM "/2(VPMM_PowerUpState_enum) -> Delay1/1
  Data Type Conversion35/1 -> [VPMM_CACPresReadyProc_flg]  "VPMM_CACPresReadyProc_flg"
  "PMM "/10(VPMM_BattHVDem_enum) -> Data Type Conversion10/1
  [VINP_ChargeWakeup_flg] -> "PMM "/15(VINP_ChargeWakeup_flg)
  [VINP_BMSHVSts_enum] -> "PMM Flag Creator "/4(VINP_BMSHVSts_enum)
  [VPMM_HVUnitSelfChkCompleted4Chrg_flg] -> "PMM "/35(VPMM_HVUnitSelfChkCompleted4Chrg_flg)
  "PMM "/23(VPMM_VCUMCUCtrlMd_enum) -> Data Type Conversion26/1
  [VPMM_PDUEACRlySta_enum] -> "PMM Flag Creator "/7(VSCP_PDUEACRlySta_enum)
  Constant31/1 -> Switch/1
  VINP_MCUFailGrade_enum/1 -> [VINP_MCUFailGrade_enum]
  [VINP_DCChrgConnectSts_enum] -> "PMM "/5(VINP_DCChrgConnectSts_enum)
  Constant71/1 -> "PMM "/69(KPMM_EHPSSpdDem_rpm)
  "PMM "/35(VPMM_ChrgPowerUpFail_flg) -> Data Type Conversion20/1
  "PMM "/8(VPMM_IRCRlyClose_flg) -> Data Type Conversion8/1
  VPSA_AlcLockPass_flg/1 -> [VPSA_AlcLockPass_flg]
  [VACC_CACPresReady_flg] -> "PMM "/1(VACC_CACPresReady_flg)
  Constant23/1 -> "PMM "/52(KPMM_TargetEnDischrgVolt_V)
  [VINP_ChargeWakeup_flg] -> PMM State Change Configuration/2(VINP_ChargeWakeup_flg)
  Data Type Conversion24/1 -> VPMM_PowerUpComplete_flg/1  "VPMM_PowerUpComplete_flg"
  [VPMM_RlyOpenCheck_flg] -> "PMM "/3(VPMM_RlyOpenCheck_flg)
  Data Type Conversion39/1 -> VPMM_PMMEHPSEnableDem_flg/1  "VPMM_PMMEHPSEnableDem_flg"
  "PMM "/7(VPMM_ChrgFault_enum) -> Data Type Conversion7/1
  Data Type Conversion25/1 -> VPMM_ExtTorquePrevent_enum/1  "VPMM_ExtTorquePrevent_enum"
  Detect Increase1/1 -> "PMM "/47(VPMM_SSBrisdetect_flg)
  VDMM_LostComMCUSta2_flg/1 -> [VDMM_LostComMCUSta2_flg]
  Switch/1 -> Detect Increase/1
  [VINP_HVPwrOffReq_enum] -> "PMM "/16(VINP_HVPwrOffReq_enum)
  [VINP_DCDCEnableStstus_enum] -> "PMM "/10(VINP_DCDCEnableStatus_enum)
  Data Type Conversion34/1 -> [VPMM_EHPSEnableProc_flg]  "VPMM_EHPSEnableProc_flg"
  "PMM "/22(VPMM_ExtTorquePrevent_enum) -> Data Type Conversion25/1
  [VINP_EHPSEnableStstus_enum] -> "PMM "/11(VINP_EHPSEnableStatus_enum)
  [VINP_BMSChrgStatus_enum] -> "PMM "/14(VINP_BMSChrgStatus_enum)
  Constant9/1 -> "PMM "/23(KPMM_ACMainRlyUpFailtime_s)
  [VINP_PushButton_flg] -> "PMM "/45(VINP_PushButton_flg), Detect Increase1/1
  Constant2/1 -> "PMM "/30(KPMM_SysInitialTO_s)
  [VPMM_PDUDCDCRlySta_enum] -> "PMM "/6(VPMM_PDUDCDCRlySta_enum)
  Data Type Conversion4/1 -> VPMM_ChrgState_enum/1  "VPMM_ChrgState_enum"
  "PMM "/28(VPMM_EHPSEnableProc_flg) -> Data Type Conversion34/1
  Constant17/1 -> "PMM "/26(KPMM_MCUDisChrgFailtime_s)
  Constant16/1 -> "PMM "/25(KPMM_BattDownFailtime_s)
  "PMM "/11(VPMM_DCDCRlyDem_enum) -> Data Type Conversion11/1
  "PMM "/5(VPMM_PowerUpFault_enum) -> Data Type Conversion5/1
  Constant25/1 -> "PMM "/31(KPMM_WaitForAfterrunFail_s)
  Constant4/1 -> "PMM "/20(KPMM_BattUpFailtime_s)
  [task_time_s] -> "PMM "/57(task_time_s)
  [VINP_PDUACRlySta_enum] -> "PMM "/49(VINP_PDUACRlySta_enum)
  Constant46/1 -> "PMM "/62(KPMM_MCUDisableFailtime_s)
  Constant59/1 -> "PMM "/66(KPMM_AlcLockCheckFailtime_s)
  Constant22/1 -> "PMM "/28(KPMM_TargetDchrgVolt_V)
  Constant18/1 -> "PMM "/38(KPMM_DCDCRlyDemDelayTime_s)
  "PMM Flag Creator "/14(VPMM_MCUHVLoopDem_enum) -> VPMM_MCUHVLoopDem_enum/1
  Constant7/1 -> "PMM "/22(KPMM_DCDCEnableFailtime_s)
  VINP_PDUMCUPosRlySta_enum/1 -> [VINP_PDUMCUPosRlySta_enum]
  Data Type Conversion22/1 -> VPMM_PowerUpInhibit_flg/1  "VPMM_PowerUpInhibit_flg"
  [VPMM_Boot2Initialize_flg] -> "PMM "/74(VPMM_Boot2Initialize_flg)
  [VPMM_AfterRun2Initialize_flg] -> "PMM "/75(VPMM_AfterRun2Initialize_flg)
  [VPMM_Initialize2Idle_flg] -> "PMM "/76(VPMM_Initialize2Idle_flg)
  [VPMM_Initialize2Charge_flg] -> "PMM "/77(VPMM_Initialize2Charge_flg)
  [VPMM_Initialize2PowerUp_flg] -> "PMM "/78(VPMM_Initialize2PowerUp_flg)
  [VPMM_PowerUp2PowerDown_flg] -> "PMM "/79(VPMM_PowerUp2PowerDown_flg)
  [VPMM_Drive2PowerDown_flg] -> "PMM "/80(VPMM_Drive2PowerDown_flg)
  [VPMM_Charge2PowerDown_flg] -> "PMM "/81(VPMM_Charge2PowerDown_flg)
  VDMM_NoFeedBack_flg/1 -> [VDMM_NoFeedBack_flg]
  VDMM_HVRlyNoFeedBack_flg/1 -> [VDMM_HVRlyNoFeedBack_flg]
  VDMM_DTCVCUPowerVolLow_flg/1 -> [VDMM_DTCVCUPowerVolLow_flg]
  VDMM_DTCVCUPowerVolHigh_flg/1 -> [VDMM_DTCVCUPowerVolHigh_flg]
  [VDMM_NoFeedBack_flg] -> PMM State Change Configuration/9(VDMM_NoFeedBack_flg)
  [VPMM_HVRlyNoFeedBack_flg] -> PMM State Change Configuration/10(VPMM_HVRlyNoFeedBack_flg)
  [VDMM_DTCVCUPowerVolHigh_flg] -> PMM State Change Configuration/11(VDMM_DTCVCUPowerVolHigh_flg)
  [VDMM_DTCVCUPowerVolLow_flg] -> PMM State Change Configuration/12(VDMM_DTCVCUPowerVolLow_flg)
  VDMM_DTCHVILWireFailure_flg/1 -> [VDMM_DTCHVILWireFailure_flg]
  [VDMM_DTCHVILWireFailure_flg] -> PMM State Change Configuration/13(VDMM_DTCHVILWireFailure_flg)
  "PMM Flag Creator "/15(VPMM_HVRlyNoFeedBack_flg) -> [VPMM_HVRlyNoFeedBack_flg]
  [VDMM_HVRlyNoFeedBack_flg] -> "PMM Flag Creator "/38(VDMM_HVRlyNoFeedBack_flg)
  [VDMM_DTCAlcLockWireFailure_flg] -> "PMM Flag Creator "/39(VDMM_DTCAlcLockWireFailure_flg)
  VDMM_DTCAlcLockWireFailure_flg/1 -> [VDMM_DTCAlcLockWireFailure_flg]
  VDMM_ProhibitCharge_flg/1 -> [VDMM_ProhibitCharge_flg]
  [VDMM_ProhibitCharge_flg] -> PMM State Change Configuration/14(VDMM_ProhibitCharge_flg)
  VDMM_ProhibitPowerUp_flg/1 -> [VDMM_ProhibitPowerUp_flg]
  [VDMM_ProhibitPowerUp_flg] -> PMM State Change Configuration/15(VDMM_ProhibitPowerUp_flg)
  VDMM_MCUForceDisable_flg/1 -> [VDMM_MCUForceDisable_flg]
  [VDMM_MCUForceDisable_flg] -> "PMM Flag Creator "/40(VDMM_MCUForceDisable_flg)
  [VPMM_SysPowerMode_enum] -> "PMM Flag Creator "/41(VPMM_SysPowerMode_enum)
  VDMM_DTCIRCS2GWireFailure_flg/1 -> [VDMM_DTCIRCS2GWireFailure_flg]
  VDMM_DTCIGNS2GWireFailure_flg/1 -> [VDMM_DTCIGNS2GWireFailure_flg]
  [VDMM_DTCIRCS2GWireFailure_flg] -> "PMM Flag Creator "/42(VDMM_DTCIRCS2GWireFailure_flg)
  [VDMM_DTCIGNS2GWireFailure_flg] -> "PMM Flag Creator "/43(VDMM_DTCIGNS2GWireFailure_flg)
  "PMM Flag Creator "/16(VPMM_IRCRlyCloseOut_flg) -> VPMM_IRCRlyClose_flg/1
  "PMM Flag Creator "/17(VPMM_IGNRlyCloseOut_flg) -> VPMM_IGNRlyClose_flg/1
  VDMM_DTCMCUCtrlMdNoFB_flg/1 -> [VDMM_DTCMCUCtrlMdNoFB_flg]
  [VDMM_DTCMCUCtrlMdNoFB_flg] -> "PMM Flag Creator "/44(VDMM_DTCMCUCtrlMdNoFB_flg)
  Data Type Conversion11/1 -> VPMM_DCDCRlyDem_enum/1  "VPMM_DCDCRlyDem_enum"
  VDMM_DTCBMSRlyNoFB_flg/1 -> [VDMM_DTCBMSRlyNoFB_flg]
  [VDMM_DTCMCUCtrlMdNoFB_flg] -> "PMM "/82(VDMM_DTCMCUCtrlMdNoFB_flg)
  [VDMM_DTCBMSRlyNoFB_flg] -> "PMM "/83(VDMM_DTCBMSRlyNoFB_flg)
  VDMM_WireFailure_flg/1 -> [VDMM_WireFailure_flg]
  [VDMM_WireFailure_flg] -> PMM State Change Configuration/16(VDMM_WireFailure_flg)
  [VSCP_LVchrgSvrMode_flg] -> PMM State Change Configuration/17(VSCP_LVchrgSvrMode_flg)
  PMM State Change Configuration/9(VPMM_LVChrgIinit2Idle_flg) -> [VPMM_LVChrgIinit2Idle_flg]
  [VINP_ParkBrakeSW_flg] -> PMM State Change Configuration/18(VINP_ParkBrakeSW_flg)
  [VINP_B2VSOC_pct] -> PMM State Change Configuration/19(VINP_B2VSOC_pct)
  VINP_ParkBrakeSW_flg/1 -> [VINP_ParkBrakeSW_flg]
  VINP_B2VSOC_pct/1 -> [VINP_B2VSOC_pct]
  [VPMM_LVChrgIinit2Idle_flg] -> "PMM Flag Creator "/45(VPMM_LVChrgIinit2Idle_flg)
  PMM State Change Configuration/10(VPMM_LVChrgInit2PowerUp_flg) -> [VPMM_LVChrgInit2PowerUp_flg]
  [VPMM_LVChrgPreActFinished_flg] -> "PMM "/84(VPMM_LVChrgPreActFinished_flg)
  [VPMM_LVChrgInit2PowerUp_flg] -> "PMM "/85(VPMM_LVChrgInit2PowerUp_flg)
  "PMM Flag Creator "/21(VPMM_TrigBrkLamp_flg) -> VPMM_TrigBrkLamp_flg/1
  "PMM Flag Creator "/20(VPMM_TrigRLamp_flg) -> VPMM_TrigRLamp_flg/1
  "PMM Flag Creator "/19(VPMM_TrigRBuzeer_flg) -> VPMM_TrigRBuzeer_flg/1
  [VPMM_SysPowerMode_enum] -> PMM State Change Configuration/20(VPMM_SysPowerMode_enum)
  [VINP_B2VSOC_pct] -> "PMM Flag Creator "/46(VINP_B2VSOC_pct)
  [VPMM_DCDCEnableDem_flg] -> "PMM Flag Creator "/47(VPMM_DCDCEnableDem_flg)
  "PMM Flag Creator "/22(VPMM_PMMDCDCEnableDem_flg) -> VPMM_PMMDCDCEnableDem_flg/1
  "PMM Flag Creator "/23(VPMM_LVChrgFinished_flg) -> [VPMM_LVChrgFinished_flg]
  [VPMM_LVChrgFinished_flg] -> PMM State Change Configuration/21(VPMM_LVChrgFinished_flg)
  "PMM Flag Creator "/24(VPMM_LVChrgDCDCDis_flg) -> [VPMM_LVChrgDCDCDis_flg]
  [VPMM_LVChrgDCDCDis_flg] -> "PMM "/86(VPMM_LVChrgDCDCDis_flg)
  Delay/1 -> [VPMM_SysPowerMode_enum]
  [VPMM_LVChrgFinished_flg] -> "PMM "/87(VPMM_LVChrgFinished_flg)
  "PMM Flag Creator "/25(VPMM_DCDCVolLowTO_flg) -> VPMM_DCDCVolLowTO_flg/1
  [VPMM_LVChrgInit2PowerUp_flg] -> "PMM Flag Creator "/48(VPMM_LVChrgInit2PowerUp_flg)
  [VPMM_PowerUpState_enum] -> PMM State Change Configuration/22(VPMM_PowerUpState_enum)
  Delay1/1 -> Data Type Conversion2/1
  [VINP_ParkBrakeSW_flg] -> "PMM "/88(VINP_ParkBrakeSW_flg)
  VINP_VCUBattVol_v/1 -> [VINP_VCUBattVol_v]
  [VINP_VCUBattVol_v] -> "PMM "/89(VINP_VCUBattVol_v)
  "PMM Flag Creator "/26(VPMM_LongIdleDetFinsh_flg) -> VPMM_LongIdleDetFinsh_flg/1
  [VTQD_GearActualPosn_enum] -> "PMM Flag Creator "/49(VTQD_GearActualPosn_enum)
  [VINP_EBSBrakeSw_enum] -> "PMM Flag Creator "/50(VINP_EBSBrakeSw_enum)
  [VINP_MotorSpd_rpm] -> "PMM Flag Creator "/51(VINP_MotorSpd_rpm)
  [VSCP_FRDoorOPSta_flg] -> "PMM Flag Creator "/52(VSCP_FRDoorOPSta_flg)
  [VSCP_MDDoorOPSta_flg] -> "PMM Flag Creator "/53(VSCP_MDDoorOPSta_flg)
  [VSCP_TDDoorOPSta_flg] -> "PMM Flag Creator "/54(VSCP_TDDoorOPSta_flg)
  VTQD_GearActualPosn_enum/1 -> [VTQD_GearActualPosn_enum]
  VINP_EBSBrakeSw_enum/1 -> [VINP_EBSBrakeSw_enum]
  VINP_MotorSpd_rpm/1 -> [VINP_MotorSpd_rpm]
  "PMM Flag Creator "/27(VPMM_LongIdle_flg) -> [VPMM_LongIdle_flg]
  [VPMM_LongIdle_flg] -> PMM State Change Configuration/23(VPMM_LongIdle_flg)
  VTQD_ActTDDoorOPSta_flg/1 -> [VSCP_TDDoorOPSta_flg]
  VTQD_ActMDDoorOPSta_flg/1 -> [VSCP_MDDoorOPSta_flg]
  VTQD_ActFRDoorOPSta_flg/1 -> [VSCP_FRDoorOPSta_flg]
  Unit Delay/1 -> PMM_SCP/1(VPMM_CACRlyDem_enum)
  [VPMM_CACRlyDem_enum] -> Unit Delay/1
  Unit Delay1/1 -> PMM_SCP/2(VPMM_EHPSRlyDem_enum)
  [VPMM_EHPSRlyDem_enum] -> Unit Delay1/1
  PMM_SCP/1(VPMM_PDUDCDCRlySta_enum) -> [VPMM_PDUDCDCRlySta_enum]
  PMM_SCP/3(VPMM_PDUEHPSRlySta_enum) -> [VPMM_PDUEHPSRlySta_enum]
  PMM_SCP/2(VPMM_PDUEACRlySta_enum) -> [VPMM_PDUEACRlySta_enum]
  VINP_PDU3in1RlySta_enum/1 -> [VINP_PDU3in1RlySta_enum]
  [VINP_PDU3in1RlySta_enum] -> PMM_SCP/3(VINP_PDU3in1RlySta_enum)
  [VINP_PDUMCUPosRlySta_enum] -> PMM_SCP/4(VINP_PDUMCUPosRlySta_enum)
  [VINP_PDUACRlySta_enum] -> PMM_SCP/5(VINP_PDUACRlySta_enum)
  PMM_SCP/4(VPMM_V2BLifeSig_cnt) -> VPMM_V2BLifeSig_cnt/1
  PMM_SCP/5(VPMM_V2BAux1OnOff_enum) -> VPMM_V2BAux1OnOff_enum/1
  PMM_SCP/6(VPMM_V2BAux2OnOff_enum) -> VPMM_V2BAux2OnOff_enum/1
  PMM_SCP/7(VPMM_V2BAux3OnOff_enum) -> VPMM_V2BAux3OnOff_enum/1
  PMM_SCP/8(VPMM_V2BMainPosRlySta_enum) -> VPMM_V2BMainPosRlySta_enum/1
  PMM_SCP/9(VPMM_V2BMainPosRlyFit_enum) -> VPMM_V2BMainPosRlyFit_enum/1
  PMM_SCP/10(VPMM_V2BACPosRlySta_enum) -> VPMM_V2BACPosRlySta_enum/1
  PMM_SCP/11(VPMM_V2BACPosRlyFit_enum) -> VPMM_V2BACPosRlyFit_enum/1
  PMM_SCP/12(VPMM_V2BAirPosRlySta_enum) -> VPMM_V2BAirPosRlySta_enum/1
  PMM_SCP/13(VPMM_V2BAirPosRlyFit_enum) -> VPMM_V2BAirPosRlyFit_enum/1
  PMM_SCP/14(VPMM_V2BOilPosRlySta_enum) -> VPMM_V2BOilrPosRlySta_enum/1
  PMM_SCP/15(VPMM_V2BOilPosRlyFit_enum) -> VPMM_V2BOilPosRlyFit_enum/1
  PMM_SCP/16(VPMM_V2BDCDCPosRlySta_enum) -> VPMM_V2BDCDCPosRlySta_enum/1
  PMM_SCP/17(VPMM_V2BDCDCPosRlyFit_enum) -> VPMM_V2BDCDCPosRlyFit_enum/1
  PMM_SCP/18(VPMM_V2BAux1RlySta_enum) -> VPMM_V2BAux1RlySta_enum/1
  PMM_SCP/19(VPMM_V2BAux1RlyFit_enum) -> VPMM_V2BAux1RlyFit_enum/1
  PMM_SCP/20(VPMM_V2BAux2RlySta_enum) -> VPMM_V2BAux2RlySta_enum/1
  PMM_SCP/21(VPMM_V2BAux2RlyFit_enum) -> VPMM_V2BAux2RlyFit_enum/1
  PMM_SCP/22(VPMM_V2BAux3RlySta_enum) -> VPMM_V2BAux3RlySta_enum/1
  PMM_SCP/23(VPMM_V2BAux3RlyFit_enum) -> VPMM_V2BAux3RlyFit_enum/1
  PMM_SCP/24(VPMM_V2BAux4RlySta_enum) -> VPMM_V2BAux4RlySta_enum/1
  PMM_SCP/25(VPMM_V2BAux4RlyFit_enum) -> VPMM_V2BAux4RlyFit_enum/1
  PMM_SCP/26(VPMM_V2BRsv1_cnt) -> VPMM_V2BRsv1_cnt/1
  PMM_SCP/27(VPMM_V2BRsv2_cnt) -> VPMM_V2BRsv2_cnt/1
  PMM_SCP/28(VPMM_VCULife1_cnt) -> VPMM_VCULife1_cnt/1
  PMM_SCP/29(VPMM_VCULife2_cnt) -> VPMM_VCULife2_cnt/1
  PMM_SCP/30(VPMM_VSPFunc_enum) -> VPMM_VSPFunc_enum/1
  PMM_SCP/31(VPMM_VSPIGNKeySta_enum) -> VPMM_VSPIGNKeySta_enum/1
  PMM_SCP/32(VPMM_VSPReversed_flg) -> VPMM_VSPReversed_flg/1
  PMM_SCP/33(VPMM_VSPTurnRight_enum) -> VPMM_VSPTurnRight_enum/1
  PMM_SCP/34(VPMM_VSPTurnLeft_enum) -> VPMM_VSPTurnLeft_enum/1
  [VPSA_Keystatus_enum] -> PMM_SCP/6(VPSA_Keystatus_enum)
  PMM_SCP/35(VPMM_AlcLockSta_enum) -> VPMM_AlcLockSta_flg/1
  [VPSA_AlcLockPass_flg] -> PMM_SCP/7(VPSA_AlcLockPass_flg)
  PMM_SCP/36(VPMM_FogTMSRlyCMD_enum) -> VPMM_FogTMSRlyCMD_enum/1
  [VINP_TransReqGear_enum] -> PMM_SCP/8(VINP_TransReqGear_enum)
  VINP_TransReqGear_enum/1 -> [VINP_TransReqGear_enum]
  [VINP_B2VPackCurr_A] -> PMM_SCP/9(VINP_B2VPackCurr_A)
  [VINP_B2VPackInsideVol_V] -> PMM_SCP/10(VINP_B2VPackInsideVol_V)
  PMM_SCP/37(VPMM_DCCurr_A) -> VPMM_DCCurr_A/1
  PMM_SCP/38(VPMM_DCVol_V) -> VPMM_DCVol_V/1
  VINP_B2VPackCurr_A/1 -> [VINP_B2VPackCurr_A]
  VINP_B2VPackInsideVol_V/1 -> [VINP_B2VPackInsideVol_V]
  Constant34/1 -> Detect Increase2/1
  Detect Increase2/1 -> "PMM "/90(KPSA_FakeWakeRESETRising_flg)
  [task_time_s] -> PMM_SCP/11(task_time_s)
